simulink model "uniciclo_FL"  (R2020a)
settings: Solver=VariableStepAuto  StartTime=0.0  StopTime=10.0  RelTol=1e-3
settings Model: Creator=Andrea_Ferroni  LastModifiedBy=Andrea_Ferroni

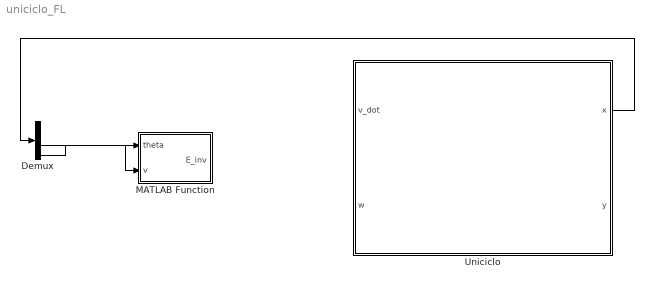
== system uniciclo_FL ==
  Demux : Demux
  MATLAB Function : MATLAB Function  TreatAsAtomicUnit=on
  Uniciclo : Subsystem
  wires:
  Uniciclo/1(x) -> Demux/1
  Demux/3 -> MATLAB Function/2(v)
  Demux/4 -> MATLAB Function/1(theta)

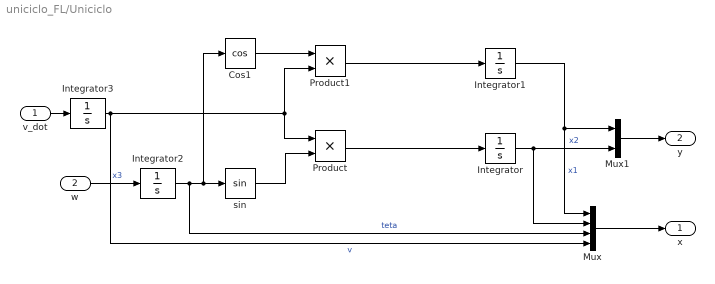
== system uniciclo_FL/Uniciclo ==
  v_dot : Inport
  w : Inport  Port=2
  Cos1 : Trigonometry  Operator=cos
  Integrator : Integrator
  Integrator1 : Integrator
  Integrator2 : Integrator  InitialCondition=pi/2
  Integrator3 : Integrator  InitialCondition=pi/2
  Mux : Mux
  Mux1 : Mux  Inputs=2
  Product : Product
  Product1 : Product
  sin : Trigonometry
  x : Outport
  y : Outport  Port=2
  wires:
  v_dot/1 -> Integrator3/1
  Cos1/1 -> Product1/1
  Product1/1 -> Integrator1/1
  Product/1 -> Integrator/1
  w/1 -> Integrator2/1  "x3"
  Integrator2/1 -> Mux/3, Cos1/1, sin/1  "teta"
  sin/1 -> Product/2
  Mux/1 -> x/1
  Integrator1/1 -> Mux/1, Mux1/1  "x1"
  Integrator/1 -> Mux/2, Mux1/2  "x2"
  Mux1/1 -> y/1
  Integrator3/1 -> Mux/4, Product1/2, Product/1  "v"

== matlab function uniciclo_FL/MATLAB Function ==
  data: theta input; v input; E_inv output
function E_inv = inv_E(theta, v)
E = [cos(theta) -v*sin(theta);
	 sin(theta)  v*cos(theta)];
E_inv = inv(E);
